simulink model "Matlab Simulink  Fig_10"  (R2022b)
settings: Solver=ode45  StartTime=0.0  StopTime=2  RelTol=1e-3  EnableMultiTasking=on
libraries: spsIGBTDiodeLib x18, spsSeriesRLCBranchLib x10, spsCurrentMeasurementLib x4, spsDCVoltageSourceLib x4, spsVoltageMeasurementLib x4, spspowerguiLib x2
settings Model: Creator=dhanu  LastModifiedBy=dell
settings SolverCC: AlgebraicLoopSolver=TrustRegion
settings DataIOCC: LimitDataPoints=on  SaveFormat=Array  ReturnWorkspaceOutputs=off
settings OptimizationCC: LifeSpan=inf
settings DebuggingCC: UnderspecifiedInitializationDetection=Classic  MergeDetectMultiDrivingBlocksExec=none  SolverPrmCheckMsg=warning  UnconnectedInputMsg=warning  UnconnectedOutputMsg=warning  UnconnectedLineMsg=warning  StateNameClashWarn=warning  SFUnexpectedBacktrackingDiag=warning  SFNoUnconditionalDefaultTransitionDiag=warning  SFExecutionAtInitializationDiag=none  SFMachineParentedDataDiag=warning  ArithmeticOperatorsInVariantConditions=warning
settings HardwareCC: ProdBitPerPointer=32  ProdBitPerSizeT=32  ProdBitPerPtrDiffT=32  ProdLargestAtomicFloat=None  ProdIntDivRoundTo=Undefined  ProdEndianess=Unspecified  ProdWordSize=32  ProdHWDeviceType=32-bit Generic
settings ModelReferenceCC: PropagateSignalLabelsOutOfModel=off
settings SFSimCC: SimUseLocalCustomCode=off  CustomCodeUndefinedFunction=UseInterfaceOnly
settings RTWCC: RTWUseLocalCustomCode=off
settings CodeAppCC: StateflowObjectComments=on
settings GRTTargetCC: TargetLangStandard=C89/C90 (ANSI)
settings ConfigComp: CovMetricSettings=dw  CovSaveCumulativeToWorkspaceVar=on  CovSaveSingleToWorkspaceVar=on  CovExternalEMLEnable=off
settings SimscapeCC: SimscapeNormalizeSystem=off

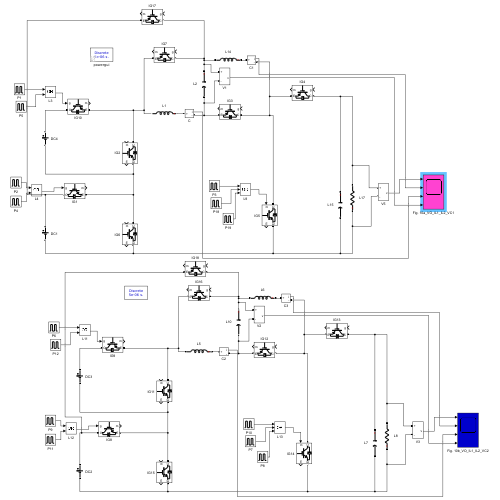
[thumbnail: Simulink's stored preview of the top-level diagram]
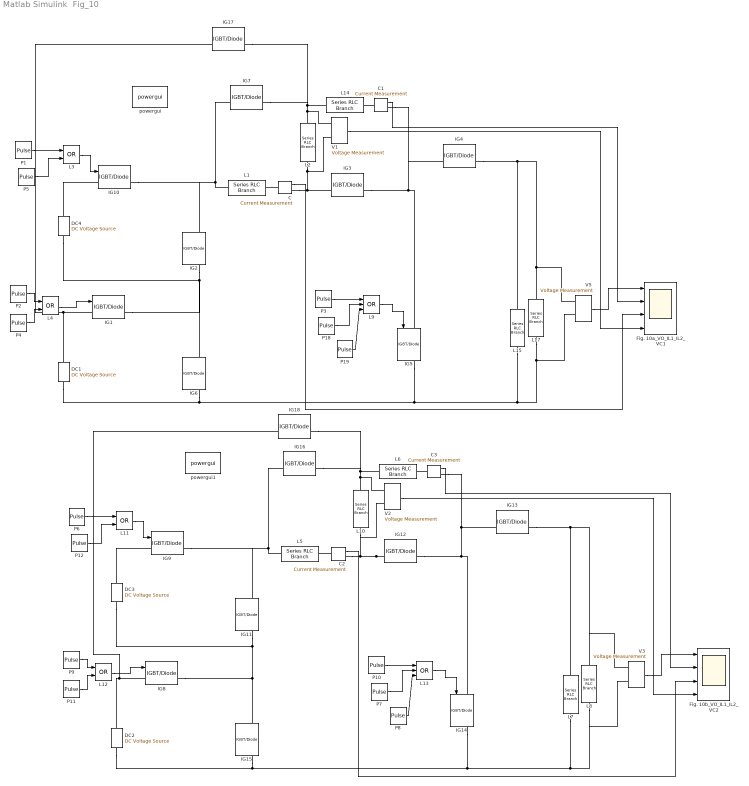
== system Matlab Simulink  Fig_10 ==
  C{,1..3} (4 alike) : spsCurrentMeasurementLib/Current Measurement  PhasorSimulation=off  OutputType=Complex  PSBequivalent=0
  DC1 : spsDCVoltageSourceLib/DC Voltage Source  Amplitude=15  Measurements=None
  DC2 : spsDCVoltageSourceLib/DC Voltage Source  Amplitude=10  Measurements=None
  DC3 : spsDCVoltageSourceLib/DC Voltage Source  Amplitude=20  Measurements=None
  DC4 : spsDCVoltageSourceLib/DC Voltage Source  Amplitude=25  Measurements=None
  Fig. 10a_VO_IL1_IL2_VC1 : Scope  NumInputPorts=4
  Fig. 10b_VO_IL1_IL2_VC2 : Scope  NumInputPorts=4
  IG{1..18} (18 alike) : spsIGBTDiodeLib/IGBT//Diode  Ron=1e-3  Rs=1e5  Cs=inf  Measurements=on
  L{1,5..6,14} (4 alike) : spsSeriesRLCBranchLib/Series RLC Branch  LConnTagsString=__new0  RConnTagsString=__new0  BranchType=L  Resistance=1  Inductance=4e-3  SetiL0=off  InitialCurrent=0  Capacitance=1e-6  Setx0=off  InitialVoltage=0  Measurements=None
  L10 : spsSeriesRLCBranchLib/Series RLC Branch  LConnTagsString=__new0  RConnTagsString=__new0  BranchType=C  Resistance=1  Inductance=1e-3  SetiL0=off  InitialCurrent=0  Capacitance=360e-6  Setx0=off  InitialVoltage=0  Measurements=None
  L{3..4,11..12} (4 alike) : Logic  Operator=OR  AllPortsSameDT=off  OutDataTypeStr=boolean
  L13 : Logic  Operator=OR  Inputs=3  AllPortsSameDT=off  OutDataTypeStr=boolean
  L15 : spsSeriesRLCBranchLib/Series RLC Branch  LConnTagsString=__new0  RConnTagsString=__new0  BranchType=C  Resistance=1  Inductance=1e-3  SetiL0=off  InitialCurrent=0  Capacitance=370e-6  Setx0=off  InitialVoltage=0  Measurements=None
  L17 : spsSeriesRLCBranchLib/Series RLC Branch  LConnTagsString=__new0  RConnTagsString=__new0  BranchType=R  Resistance=80  Inductance=1e-3  SetiL0=off  InitialCurrent=0  Capacitance=1000e-6  Setx0=off  InitialVoltage=0  Measurements=None
  L2 : spsSeriesRLCBranchLib/Series RLC Branch  LConnTagsString=__new0  RConnTagsString=__new0  BranchType=C  Resistance=1  Inductance=1e-3  SetiL0=off  InitialCurrent=0  Capacitance=360e-6  Setx0=off  InitialVoltage=0  Measurements=None
  L7 : spsSeriesRLCBranchLib/Series RLC Branch  LConnTagsString=__new0  RConnTagsString=__new0  BranchType=C  Resistance=1  Inductance=1e-3  SetiL0=off  InitialCurrent=0  Capacitance=470e-6  Setx0=off  InitialVoltage=0  Measurements=None
  L8 : spsSeriesRLCBranchLib/Series RLC Branch  LConnTagsString=__new0  RConnTagsString=__new0  BranchType=R  Resistance=80  Inductance=1e-3  SetiL0=off  InitialCurrent=0  Capacitance=1000e-6  Setx0=off  InitialVoltage=0  Measurements=None
  L9 : Logic  Operator=OR  Inputs=3  AllPortsSameDT=off  OutDataTypeStr=boolean
  P1 : DiscretePulseGenerator  PulseType=Time based  Amplitude=15  Period=1/10000  PulseWidth=30
  P10 : DiscretePulseGenerator  PulseType=Time based  Amplitude=15  Period=1/10000  PulseWidth=20
  P11 : DiscretePulseGenerator  PulseType=Time based  Amplitude=15  Period=1/10000  PulseWidth=20  PhaseDelay=0.000021
  P12 : DiscretePulseGenerator  PulseType=Time based  Amplitude=15  Period=1/10000  PulseWidth=20  PhaseDelay=0.000021
  P18 : DiscretePulseGenerator  PulseType=Time based  Amplitude=15  Period=1/10000  PulseWidth=30  PhaseDelay=0.000031
  P19 : DiscretePulseGenerator  PulseType=Time based  Amplitude=15  Period=1/10000  PulseWidth=10  PhaseDelay=0.000061
  P2 : DiscretePulseGenerator  PulseType=Time based  Amplitude=15  Period=1/10000  PulseWidth=10  PhaseDelay=0.000061
  P3 : DiscretePulseGenerator  PulseType=Time based  Amplitude=15  Period=1/10000  PulseWidth=30
  P4 : DiscretePulseGenerator  PulseType=Time based  Amplitude=15  Period=1/10000  PulseWidth=30  PhaseDelay=0.000031
  P5 : DiscretePulseGenerator  PulseType=Time based  Amplitude=15  Period=1/10000  PulseWidth=30  PhaseDelay=0.000031
  P6 : DiscretePulseGenerator  PulseType=Time based  Amplitude=15  Period=1/10000  PulseWidth=20
  P7 : DiscretePulseGenerator  PulseType=Time based  Amplitude=15  Period=1/10000  PulseWidth=20  PhaseDelay=0.000021
  P8 : DiscretePulseGenerator  PulseType=Time based  Amplitude=15  Period=1/10000  PulseWidth=10  PhaseDelay=0.000041
  P9 : DiscretePulseGenerator  PulseType=Time based  Amplitude=15  Period=1/10000  PulseWidth=10  PhaseDelay=0.000051
  V{1..3,5} (4 alike) : spsVoltageMeasurementLib/Voltage Measurement  PhasorSimulation=off  OutputType=Complex  PSBequivalent=0
  powergui : spspowerguiLib/powergui  Priority=1  SimulationMode=Discrete  SampleTime=50e-7  frequency=60  Iterations=50  frequencyindice=0  Pbase=100e6  ErrMax=1e-4  UnitsV=kV  UnitsW=MW  buscounter=0  FunctionMessages=off  echomessages=off  EnableUseOfTLC=off  CurrentSourceSwitches=off  DisableSnubberDevices=off  DisableRonSwitches=off  DisableVfSwitches=off  DisplayEquations=off  AutomaticDiscreteSolvers=off  SolverType=Tustin  Interpol=off  ExternalGateDelay=off  methode=off  Ts=0  x0status=blocks  SPID=off  SwTol=0  HookPort=off  NonlinearTolerance=1e-4  nMaxIteration=100  ContinueOnMaxIteration=off  RestoreLinks=warning  ResistiveCurrentMeasurement=off  Frange=[0:2:500]  Ylog=off  Xlog=on  ShowGrid=off  save=off  variable=ZData  structure=0  ZoomFFT=off  StartTime=0.0  cycles=1  DisplayStyle=1  fundamental=60  FreqAxis=off  MaxFrequency=1000  frequencyindicesteady=1  RmsSteady=1  display=off
  powergui1 : spspowerguiLib/powergui  Priority=1  SimulationMode=Discrete  SampleTime=50e-7  frequency=60  Iterations=50  frequencyindice=0  Pbase=100e6  ErrMax=1e-4  UnitsV=kV  UnitsW=MW  buscounter=0  FunctionMessages=off  echomessages=off  EnableUseOfTLC=off  CurrentSourceSwitches=off  DisableSnubberDevices=off  DisableRonSwitches=off  DisableVfSwitches=off  DisplayEquations=off  AutomaticDiscreteSolvers=off  SolverType=Tustin  Interpol=off  ExternalGateDelay=off  methode=off  Ts=0  x0status=blocks  SPID=off  SwTol=0  HookPort=off  NonlinearTolerance=1e-4  nMaxIteration=100  ContinueOnMaxIteration=off  RestoreLinks=warning  ResistiveCurrentMeasurement=off  Frange=[0:2:500]  Ylog=off  Xlog=on  ShowGrid=off  save=off  variable=ZData  structure=0  ZoomFFT=off  StartTime=0.0  cycles=1  DisplayStyle=1  fundamental=60  FreqAxis=off  MaxFrequency=1000  frequencyindicesteady=1  RmsSteady=1  display=off
  wires:
  P1/1 -> L3/1
  L3/1 -> IG10/1
  P2/1 -> L4/1
  L4/1 -> IG1/1
  P4/1 -> L4/2
  P5/1 -> L3/2
  V5/1 -> Fig. 10a_VO_IL1_IL2_VC1/1
  C/1 -> Fig. 10a_VO_IL1_IL2_VC1/3
  V1/1 -> Fig. 10a_VO_IL1_IL2_VC1/4
  C1/1 -> Fig. 10a_VO_IL1_IL2_VC1/2
  P18/1 -> L9/2
  L9/1 -> IG5/1
  P3/1 -> L9/1
  P19/1 -> L9/3
  P8/1 -> L13/3
  L13/1 -> IG14/1
  P7/1 -> L13/2
  V2/1 -> Fig. 10b_VO_IL1_IL2_VC2/4
  L11/1 -> IG9/1
  C2/1 -> Fig. 10b_VO_IL1_IL2_VC2/3
  P6/1 -> L11/1
  C3/1 -> Fig. 10b_VO_IL1_IL2_VC2/2
  P11/1 -> L12/2
  P9/1 -> L12/1
  V3/1 -> Fig. 10b_VO_IL1_IL2_VC2/1
  P12/1 -> L11/2
  P10/1 -> L13/1
  L12/1 -> IG8/1
  connections:
  V5/LConn1 -- L17/RConn1 -- L15/LConn1 -- IG4/LConn1
  IG7/RConn1 -- IG2/LConn1 -- IG10/RConn1 -- L1/RConn1
  DC4/LConn1 -- IG2/RConn1 -- IG6/LConn1 -- IG1/RConn1
  IG1/LConn1 -- IG17/RConn1 -- DC1/RConn1
  L17/LConn1 -- IG5/RConn1 -- IG6/RConn1 -- DC1/LConn1 -- L15/RConn1 -- V5/LConn2
  IG4/RConn1 -- C1/RConn1 -- IG5/LConn1 -- IG3/LConn1
  DC4/RConn1 -- IG10/LConn1
  L14/RConn1 -- IG17/LConn1 -- IG7/LConn1 -- L2/LConn1 -- V1/LConn1
  L2/RConn1 -- C/RConn1 -- IG3/RConn1 -- V1/LConn2
  C/LConn1 -- L1/LConn1
  C1/LConn1 -- L14/LConn1
  IG12/RConn1 -- L10/RConn1 -- V2/LConn2 -- C2/RConn1
  DC2/LConn1 -- IG15/RConn1 -- IG14/RConn1 -- L8/LConn1 -- V3/LConn2 -- L7/RConn1
  IG8/RConn1 -- IG15/LConn1 -- IG11/RConn1 -- DC3/LConn1
  IG13/LConn1 -- L7/LConn1 -- V3/LConn1 -- L8/RConn1
  L5/RConn1 -- IG16/RConn1 -- IG11/LConn1 -- IG9/RConn1
  V2/LConn1 -- IG18/LConn1 -- IG16/LConn1 -- L6/RConn1 -- L10/LConn1
  C3/RConn1 -- IG13/RConn1 -- IG14/LConn1 -- IG12/LConn1
  C3/LConn1 -- L6/LConn1
  C2/LConn1 -- L5/LConn1
  DC3/RConn1 -- IG9/LConn1
  IG8/LConn1 -- IG18/RConn1 -- DC2/RConn1
